simulink model "Fly_By_Wire_Activity_Diagram"  (R2024a)
settings: Solver=VariableStepAuto  StartTime=0.0  StopTime=10.0  RelTol=1e-3
settings Model: Creator=kmara  LastModifiedBy=chico

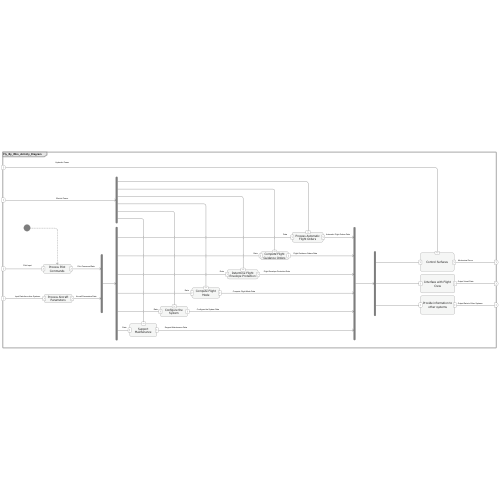
[thumbnail: Simulink's stored preview of the top-level diagram]
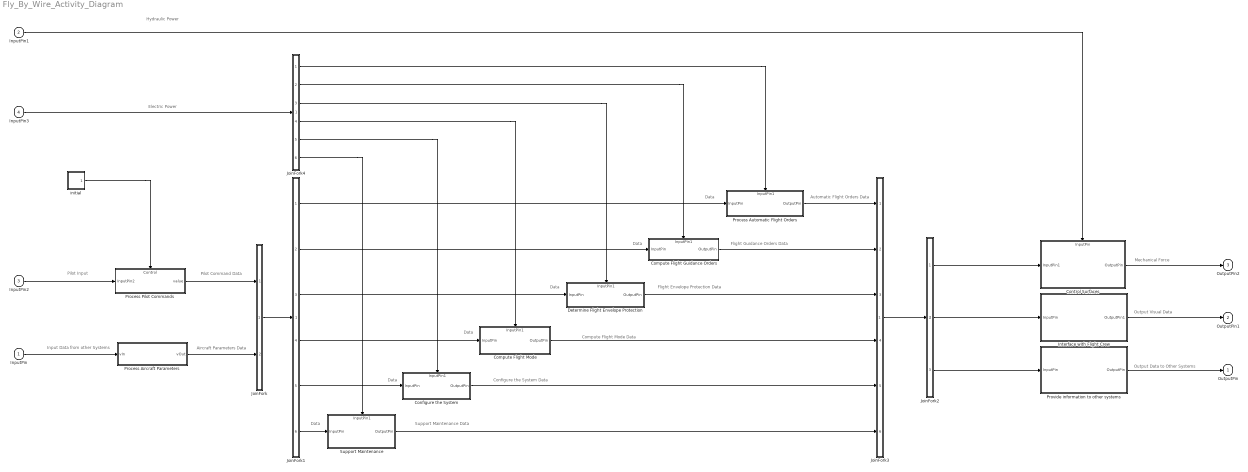
== system Fly_By_Wire_Activity_Diagram ==
  note: Data
  note: Data
  note: Data
  note: Data
  note: Data
  note: Data
  note: Flight Guidance Orders Data
  note: Support Maintenance Data
  note: Configure the System Data
  note: Compute Flight Mode Data
  note: Flight Envelope Protection Data
  note: Electric Power
  note: Hydraulic Power
  note: Mechanical Force
  note: Output Data to Other Systems
  note: Output Visual Data
  note: Aircraft Parameters Data
  note: Pilot Command Data
  note: Input Data from other Systems
  note: Pilot Input
  note: Automatic Flight Orders Data
  InputPin : Inport
  InputPin1 : Inport  Port=2
  InputPin2 : Inport  Port=3
  InputPin3 : Inport  Port=4
  Compute Flight Guidance Orders : Subsystem
      settings: CopyFcn=set_param(gcbh,'LinkStatus','none');  PortSchema="{\"entries\":[{\"content\":{\"sides\":[{\"content\":{\"connectorIds\":[\"In1\"]},\"type\":\"ConnectorPlacement.EquallySpacedRectSide\",\"uuid\":\"dc343963-6e4e-476c-b653-c476baadf41b\"},{\"content\":{\"connectorIds\":[\"Out1\"],\"side\":\"RIGHT\"},\"type\":\"ConnectorPlacement.EquallySpacedRectSide\",\"uuid\":\"f73bc494-9731-4a89-bb4e-7a23fbe62eb2\"},{\"content\":{\"connectorIds\":[\"In2\"],\"side\":\"TOP\"},\"type\":\"ConnectorPlacement.EquallySpacedRectSide\",\"uuid\":\"1e7ffc2d-9d7e-466b-bdbd-f59760556c1c\"}]},\"type\":\"ConnectorPlacement.EquallySpacedConnector\",\"uuid\":\"f6e96b6d-91af-4316-811c-753d38ee8aa9\"}],\"packageUris\":[\"http://schema.mathworks.com/mf0/Connector/R2020b\"],\"version\":\"1.0\"}"
  Compute Flight Mode : Subsystem
      settings: CopyFcn=set_param(gcbh,'LinkStatus','none');  PortSchema="{\"entries\":[{\"content\":{\"sides\":[{\"content\":{\"connectorIds\":[\"In1\"]},\"type\":\"ConnectorPlacement.EquallySpacedRectSide\",\"uuid\":\"dc343963-6e4e-476c-b653-c476baadf41b\"},{\"content\":{\"connectorIds\":[\"Out1\"],\"side\":\"RIGHT\"},\"type\":\"ConnectorPlacement.EquallySpacedRectSide\",\"uuid\":\"f73bc494-9731-4a89-bb4e-7a23fbe62eb2\"},{\"content\":{\"connectorIds\":[\"In2\"],\"side\":\"TOP\"},\"type\":\"ConnectorPlacement.EquallySpacedRectSide\",\"uuid\":\"1e7ffc2d-9d7e-466b-bdbd-f59760556c1c\"}]},\"type\":\"ConnectorPlacement.EquallySpacedConnector\",\"uuid\":\"f6e96b6d-91af-4316-811c-753d38ee8aa9\"}],\"packageUris\":[\"http://schema.mathworks.com/mf0/Connector/R2020b\"],\"version\":\"1.0\"}"
  Configure the System : Subsystem
      settings: CopyFcn=set_param(gcbh,'LinkStatus','none');  PortSchema="{\"entries\":[{\"content\":{\"sides\":[{\"content\":{\"connectorIds\":[\"In1\"]},\"type\":\"ConnectorPlacement.EquallySpacedRectSide\",\"uuid\":\"dc343963-6e4e-476c-b653-c476baadf41b\"},{\"content\":{\"connectorIds\":[\"Out1\"],\"side\":\"RIGHT\"},\"type\":\"ConnectorPlacement.EquallySpacedRectSide\",\"uuid\":\"f73bc494-9731-4a89-bb4e-7a23fbe62eb2\"},{\"content\":{\"connectorIds\":[\"In2\"],\"side\":\"TOP\"},\"type\":\"ConnectorPlacement.EquallySpacedRectSide\",\"uuid\":\"1e7ffc2d-9d7e-466b-bdbd-f59760556c1c\"}]},\"type\":\"ConnectorPlacement.EquallySpacedConnector\",\"uuid\":\"f6e96b6d-91af-4316-811c-753d38ee8aa9\"}],\"packageUris\":[\"http://schema.mathworks.com/mf0/Connector/R2020b\"],\"version\":\"1.0\"}"
  Control Surfaces : Subsystem
      settings: CopyFcn=set_param(gcbh,'LinkStatus','none');  PortSchema="{\"entries\":[{\"content\":{\"sides\":[{\"content\":{\"connectorIds\":[\"In1\"]},\"type\":\"ConnectorPlacement.EquallySpacedRectSide\",\"uuid\":\"2ddb3d2c-7641-4b68-8414-a04d5ef25b67\"},{\"content\":{\"connectorIds\":[\"Out1\"],\"side\":\"RIGHT\"},\"type\":\"ConnectorPlacement.EquallySpacedRectSide\",\"uuid\":\"f7cbdc66-1b34-432a-881d-8e1036cc0e2f\"},{\"content\":{\"connectorIds\":[\"In2\"],\"side\":\"TOP\"},\"type\":\"ConnectorPlacement.EquallySpacedRectSide\",\"uuid\":\"18c11060-a322-4914-8699-b4441c1eb626\"},{\"content\":{\"side\":\"BOTTOM\"},\"type\":\"ConnectorPlacement.EquallySpacedRectSide\",\"uuid\":\"7eb07c5e-4504-4f7e-9498-9c2c466ba7e4\"}]},\"type\":\"ConnectorPlacement.EquallySpacedConnector\",\"uuid\":\"23272bc1-2e4d-4559-8de7-ed58f314f6cf\"}],\"packageUris\":[\"http://schema.mathworks.com/mf0/Connector/R2020b\"],\"version\":\"1.0\"}"
  Determine Flight Envelope Protection : Subsystem
      settings: CopyFcn=set_param(gcbh,'LinkStatus','none');  PortSchema="{\"entries\":[{\"content\":{\"sides\":[{\"content\":{\"connectorIds\":[\"In1\"]},\"type\":\"ConnectorPlacement.EquallySpacedRectSide\",\"uuid\":\"dc343963-6e4e-476c-b653-c476baadf41b\"},{\"content\":{\"connectorIds\":[\"Out1\"],\"side\":\"RIGHT\"},\"type\":\"ConnectorPlacement.EquallySpacedRectSide\",\"uuid\":\"f73bc494-9731-4a89-bb4e-7a23fbe62eb2\"},{\"content\":{\"connectorIds\":[\"In2\"],\"side\":\"TOP\"},\"type\":\"ConnectorPlacement.EquallySpacedRectSide\",\"uuid\":\"1e7ffc2d-9d7e-466b-bdbd-f59760556c1c\"}]},\"type\":\"ConnectorPlacement.EquallySpacedConnector\",\"uuid\":\"f6e96b6d-91af-4316-811c-753d38ee8aa9\"}],\"packageUris\":[\"http://schema.mathworks.com/mf0/Connector/R2020b\"],\"version\":\"1.0\"}"
  Interface with Flight Crew : Subsystem
      settings: CopyFcn=set_param(gcbh,'LinkStatus','none');
  JoinFork : Subsystem
      settings: CopyFcn=set_param(gcbh,'LinkStatus','none');
  JoinFork1 : Subsystem
      settings: CopyFcn=set_param(gcbh,'LinkStatus','none');
  JoinFork2 : Subsystem
      settings: CopyFcn=set_param(gcbh,'LinkStatus','none');
  JoinFork3 : Subsystem
      settings: CopyFcn=set_param(gcbh,'LinkStatus','none');
  JoinFork4 : Subsystem
      settings: CopyFcn=set_param(gcbh,'LinkStatus','none');
  Process Aircraft Parameters : Subsystem
      settings: CopyFcn=set_param(gcbh,'LinkStatus','none');
  Process Automatic Flight Orders : Subsystem
      settings: CopyFcn=set_param(gcbh,'LinkStatus','none');  PortSchema="{\"entries\":[{\"content\":{\"sides\":[{\"content\":{\"connectorIds\":[\"In1\"]},\"type\":\"ConnectorPlacement.EquallySpacedRectSide\",\"uuid\":\"dc343963-6e4e-476c-b653-c476baadf41b\"},{\"content\":{\"connectorIds\":[\"Out1\"],\"side\":\"RIGHT\"},\"type\":\"ConnectorPlacement.EquallySpacedRectSide\",\"uuid\":\"f73bc494-9731-4a89-bb4e-7a23fbe62eb2\"},{\"content\":{\"connectorIds\":[\"In2\"],\"side\":\"TOP\"},\"type\":\"ConnectorPlacement.EquallySpacedRectSide\",\"uuid\":\"1e7ffc2d-9d7e-466b-bdbd-f59760556c1c\"}]},\"type\":\"ConnectorPlacement.EquallySpacedConnector\",\"uuid\":\"f6e96b6d-91af-4316-811c-753d38ee8aa9\"}],\"packageUris\":[\"http://schema.mathworks.com/mf0/Connector/R2020b\"],\"version\":\"1.0\"}"
  Process Pilot Commands : Subsystem
      settings: CopyFcn=set_param(gcbh,'LinkStatus','none');  PortSchema="{\"entries\":[{\"content\":{\"sides\":[{\"content\":{\"connectorIds\":[\"In1\"]},\"type\":\"ConnectorPlacement.EquallySpacedRectSide\",\"uuid\":\"0b06954e-1f42-4c66-80f6-50caccd35b38\"},{\"content\":{\"connectorIds\":[\"Out1\"],\"side\":\"RIGHT\"},\"type\":\"ConnectorPlacement.EquallySpacedRectSide\",\"uuid\":\"d4c7d9b4-a432-4e54-82a9-4fe0c01d1e29\"},{\"content\":{\"connectorIds\":[\"In2\"],\"side\":\"TOP\"},\"type\":\"ConnectorPlacement.EquallySpacedRectSide\",\"uuid\":\"1e21e45d-d3be-467f-971e-54d425f58506\"}]},\"type\":\"ConnectorPlacement.EquallySpacedConnector\",\"uuid\":\"2f7b3a7b-af82-4338-b5a5-09d48562ebec\"}],\"packageUris\":[\"http://schema.mathworks.com/mf0/Connector/R2020b\"],\"version\":\"1.0\"}"
  Provide information to other systems : Subsystem
      settings: CopyFcn=set_param(gcbh,'LinkStatus','none');
  Support Maintenance : Subsystem
      settings: CopyFcn=set_param(gcbh,'LinkStatus','none');  PortSchema="{\"entries\":[{\"content\":{\"sides\":[{\"content\":{\"connectorIds\":[\"In1\"]},\"type\":\"ConnectorPlacement.EquallySpacedRectSide\",\"uuid\":\"dc343963-6e4e-476c-b653-c476baadf41b\"},{\"content\":{\"connectorIds\":[\"Out1\"],\"side\":\"RIGHT\"},\"type\":\"ConnectorPlacement.EquallySpacedRectSide\",\"uuid\":\"f73bc494-9731-4a89-bb4e-7a23fbe62eb2\"},{\"content\":{\"connectorIds\":[\"In2\"],\"side\":\"TOP\"},\"type\":\"ConnectorPlacement.EquallySpacedRectSide\",\"uuid\":\"1e7ffc2d-9d7e-466b-bdbd-f59760556c1c\"}]},\"type\":\"ConnectorPlacement.EquallySpacedConnector\",\"uuid\":\"f6e96b6d-91af-4316-811c-753d38ee8aa9\"}],\"packageUris\":[\"http://schema.mathworks.com/mf0/Connector/R2020b\"],\"version\":\"1.0\"}"
  initial : Subsystem
      settings: CopyFcn=set_param(gcbh,'LinkStatus','none');
  OutputPin : Outport
  OutputPin1 : Outport  Port=2
  OutputPin2 : Outport  Port=3
  wires:
  initial/1(Control) -> Process Pilot Commands/2(Control)
  Process Pilot Commands/1(value) -> JoinFork/1(InputPin)
  Process Aircraft Parameters/1(vOut) -> JoinFork/2(InputPin1)
  JoinFork/1(Out1) -> JoinFork1/1(InputPin)
  JoinFork1/3(Out2) -> Determine Flight Envelope Protection/1(InputPin)
  JoinFork1/2(Out3) -> Compute Flight Guidance Orders/1(InputPin)
  JoinFork1/1(OutputPin) -> Process Automatic Flight Orders/1(InputPin)
  InputPin/1 -> Process Aircraft Parameters/1(vIn)
  JoinFork1/5(Out4) -> Configure the System/1(InputPin)
  JoinFork1/6(Out1) -> Support Maintenance/1(InputPin)
  Provide information to other systems/1(OutputPin) -> OutputPin/1
  InputPin1/1 -> Control Surfaces/2(InputPin)
  Control Surfaces/1(OutputPin) -> OutputPin2/1
  JoinFork1/4(Out5) -> Compute Flight Mode/1(InputPin)
  Determine Flight Envelope Protection/1(OutputPin) -> JoinFork3/3(InputPin)
  Compute Flight Mode/1(OutputPin) -> JoinFork3/4(InputPin1)
  Configure the System/1(OutputPin) -> JoinFork3/5(InputPin2)
  Support Maintenance/1(OutputPin) -> JoinFork3/6(InputPin3)
  Process Automatic Flight Orders/1(OutputPin) -> JoinFork3/1(InputPin4)
  JoinFork3/1(Out1) -> JoinFork2/1(InputPin)
  Compute Flight Guidance Orders/1(OutputPin) -> JoinFork3/2(InputPin5)
  JoinFork2/2(Out1) -> Interface with Flight Crew/1(InputPin)
  JoinFork2/3(Out2) -> Provide information to other systems/1(InputPin)
  InputPin2/1 -> Process Pilot Commands/1(InputPin2)
  Interface with Flight Crew/1(OutputPin1) -> OutputPin1/1
  InputPin3/1 -> JoinFork4/1(InputPin)
  JoinFork4/1(Out2) -> Process Automatic Flight Orders/2(InputPin1)
  JoinFork4/2(Out3) -> Compute Flight Guidance Orders/2(InputPin1)
  JoinFork4/3(Out4) -> Determine Flight Envelope Protection/2(InputPin1)
  JoinFork4/4(Out5) -> Compute Flight Mode/2(InputPin1)
  JoinFork4/5(Out6) -> Configure the System/2(InputPin1)
  JoinFork4/6(Out1) -> Support Maintenance/2(InputPin1)
  JoinFork2/1(Out3) -> Control Surfaces/1(InputPin1)

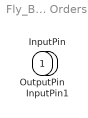
== system Fly_By_Wire_Activity_Diagram/Compute Flight Guidance Orders ==
  InputPin : Inport
  InputPin1 : Inport  Port=2
  OutputPin : Outport  OutDataTypeStr=double  PortDimensions=1

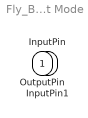
== system Fly_By_Wire_Activity_Diagram/Compute Flight Mode ==
  InputPin : Inport
  InputPin1 : Inport  Port=2
  OutputPin : Outport  OutDataTypeStr=double  PortDimensions=1

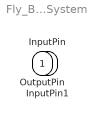
== system Fly_By_Wire_Activity_Diagram/Configure the System ==
  InputPin : Inport
  InputPin1 : Inport  Port=2
  OutputPin : Outport  OutDataTypeStr=double  PortDimensions=1

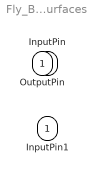
== system Fly_By_Wire_Activity_Diagram/Control Surfaces ==
  InputPin1 : Inport
  InputPin : Inport  Port=2
  OutputPin : Outport  OutDataTypeStr=double  PortDimensions=1

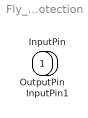
== system Fly_By_Wire_Activity_Diagram/Determine Flight Envelope Protection ==
  InputPin : Inport
  InputPin1 : Inport  Port=2
  OutputPin : Outport  OutDataTypeStr=double  PortDimensions=1

== system Fly_By_Wire_Activity_Diagram/Interface with Flight Crew ==
  InputPin : Inport
  OutputPin1 : Outport  OutDataTypeStr=double  PortDimensions=1

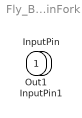
== system Fly_By_Wire_Activity_Diagram/JoinFork ==
  InputPin : Inport
  InputPin1 : Inport  Port=2
  Out1 : Outport

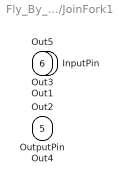
== system Fly_By_Wire_Activity_Diagram/JoinFork1 ==
  InputPin : Inport
  OutputPin : Outport  OutDataTypeStr=double  PortDimensions=1
  Out3 : Outport  Port=2
  Out2 : Outport  Port=3
  Out5 : Outport  Port=4
  Out4 : Outport  Port=5
  Out1 : Outport  Port=6

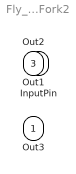
== system Fly_By_Wire_Activity_Diagram/JoinFork2 ==
  InputPin : Inport
  Out3 : Outport
  Out1 : Outport  Port=2
  Out2 : Outport  Port=3

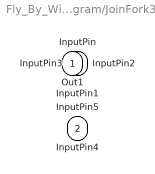
== system Fly_By_Wire_Activity_Diagram/JoinFork3 ==
  InputPin4 : Inport
  InputPin5 : Inport  Port=2
  InputPin : Inport  Port=3
  InputPin1 : Inport  Port=4
  InputPin2 : Inport  Port=5
  InputPin3 : Inport  Port=6
  Out1 : Outport

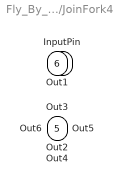
== system Fly_By_Wire_Activity_Diagram/JoinFork4 ==
  InputPin : Inport
  Out2 : Outport
  Out3 : Outport  Port=2
  Out4 : Outport  Port=3
  Out5 : Outport  Port=4
  Out6 : Outport  Port=5
  Out1 : Outport  Port=6

== system Fly_By_Wire_Activity_Diagram/Process Aircraft Parameters ==
  vIn : Inport
  vOut : Outport

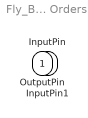
== system Fly_By_Wire_Activity_Diagram/Process Automatic Flight Orders ==
  InputPin : Inport
  InputPin1 : Inport  Port=2
  OutputPin : Outport  OutDataTypeStr=double  PortDimensions=1

== system Fly_By_Wire_Activity_Diagram/Process Pilot Commands ==
  InputPin2 : Inport
  Control : Inport  Port=2
  value : Outport

== system Fly_By_Wire_Activity_Diagram/Provide information to other systems ==
  InputPin : Inport
  OutputPin : Outport  OutDataTypeStr=double  PortDimensions=1

== system Fly_By_Wire_Activity_Diagram/Support Maintenance ==
  InputPin : Inport
  InputPin1 : Inport  Port=2
  OutputPin : Outport  OutDataTypeStr=double  PortDimensions=1

== system Fly_By_Wire_Activity_Diagram/initial ==
  Control : Outport
